simulink model "Q_1_Vibration_absorber"  (R2020b)
settings: Solver=VariableStepAuto  StartTime=0.0  StopTime=10  RelTol=1e-3
undefined symbols (not defined in the file or in its folder): b, k1, k12, M1, M2
settings Model: DataDictionary=Data_dict.sldd  Creator=Shree  LastModifiedBy=Shree

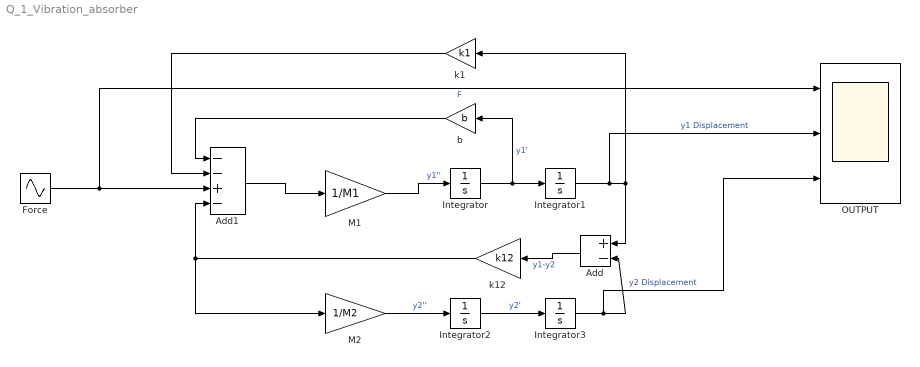
== system Q_1_Vibration_absorber ==
  Add : Sum  Inputs=+-
  Add1 : Sum  Inputs=--+-
  Force : Sin  Amplitude=2  Frequency=10  SampleTime=0
  Integrator{,1..3} (4 alike) : Integrator
  M1 : Gain  Gain=1/M1
  M2 : Gain  Gain=1/M2
  OUTPUT : Scope  NumInputPorts=3
  b : Gain  Gain=b
  k1 : Gain  Gain=k1
  k12 : Gain  Gain=k12
  wires:
  Integrator1/1 -> OUTPUT/2, k1/1, Add/1  "y1 Displacement"
  Integrator3/1 -> OUTPUT/3, Add/2  "y2 Displacement"
  Add/1 -> k12/1  "y1-y2"
  M1/1 -> Integrator/1  "y1''"
  Integrator/1 -> b/1, Integrator1/1  "y1'"
  M2/1 -> Integrator2/1  "y2''"
  Integrator2/1 -> Integrator3/1  "y2'"
  b/1 -> Add1/1
  k1/1 -> Add1/2
  k12/1 -> Add1/4, M2/1
  Add1/1 -> M1/1
  Force/1 -> OUTPUT/1, Add1/3  "F"
